simulink model "ev-pmsm-foc-model"  (R2025a)
settings: Solver=VariableStepAuto  StartTime=0.0  StopTime=10  RelTol=1e-3
undefined symbols (not defined in the file): J_m, K_d, k_g, Ki, Ki_s, Kp, Kp_s, L, lambda, p, R, r_w, T_rr
libraries: eeTransforms x4, slpidlib x3
settings Model: Creator=MEET  LastModifiedBy=MEET
settings SolverCC: ZeroCrossAlgorithm=Adaptive
settings DebuggingCC: IgnoredZcDiagnostic=none

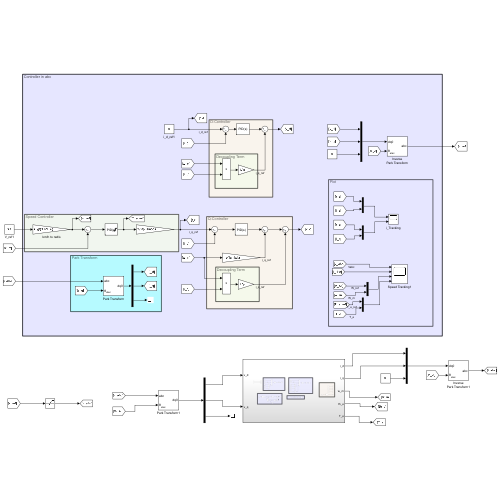
[thumbnail: Simulink's stored preview of the top-level diagram]
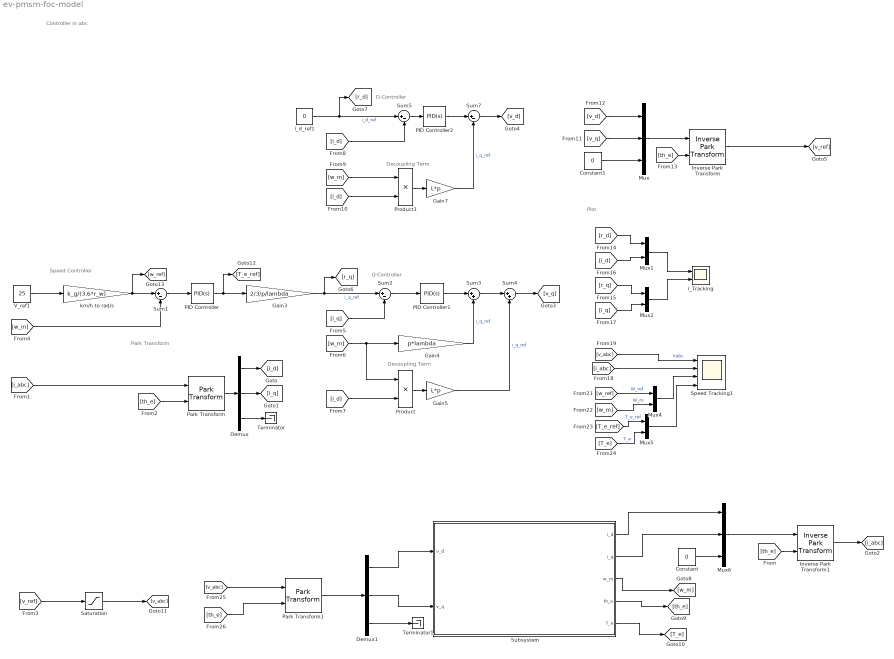
== system ev-pmsm-foc-model ==
  note: Controller in abc
  note: D-Controller
  note: Park Transform
  note: Decoupling Term
  note: Plot
  note: Decoupling Term
  note: Speed Controller
  note: Q-Controller
  Constant : Constant  Value=0
  Constant1 : Constant  Value=0
  Demux : Demux  Outputs=3
  Demux1 : Demux  Outputs=3
  Gain3 : Gain  Gain=2/3/p/lambda
  Gain4 : Gain  Gain=p*lambda
  Gain5 : Gain  Gain=L*p
  Gain7 : Gain  Gain=L*p
  Inverse Park Transform : eeTransforms/Inverse Park Transform  AxisAlignment=D-axis  PowerInvariant=off
      settings: LibrarySourceBlock=|
      | ee_sl_lib/Mathematical
      | Transforms/Inverse
      | Park Transform
  Inverse Park Transform1 : eeTransforms/Inverse Park Transform  AxisAlignment=D-axis  PowerInvariant=off
      settings: LibrarySourceBlock=|
      | ee_sl_lib/Mathematical
      | Transforms/Inverse
      | Park Transform
  Mux : Mux  Inputs=3
  Mux{1..2,4..5} (4 alike) : Mux  Inputs=2
  Mux6 : Mux  Inputs=3
  PID Controller : slpidlib/PID Controller  Controller=PID  Form=Parallel  TimeDomain=Continuous-time  UseExternalTs=off  SampleTime=-1  IntegratorMethod=Forward Euler  FilterMethod=Forward Euler  ControllerParametersSource=internal  P=Kp_s  I=Ki_s  UseKiTs=off  D=0  UseExternalDerivativeSource=off  N=100  UseFilter=on  TunerSelectOption=Transfer Function Based (PID Tuner App)  InitialConditionSource=internal  InitialConditionForIntegrator=0  InitialConditionForFilter=0  DifferentiatorICPrevScaledInput=0  ExternalReset=none  TrackingMode=off  Kt=1  LimitOutput=on  SatLimitsSource=internal  UpperSaturationLimit=108  LowerSaturationLimit=-108  LinearizeAsGain=on  AntiWindupMode=clamping  Kb=1  LimitIntegrator=off  UpperIntegratorSaturationLimit=inf  LowerIntegratorSaturationLimit=-inf  POutMin=[]  POutMax=[]  IOutMin=[]  IOutMax=[]  DOutMin=[]  DOutMax=[]  NOutMin=[]  NOutMax=[]  SumOutMin=[]  SumOutMax=[]  SaturationOutMin=[]  SaturationOutMax=[]  PParamMin=[]  PParamMax=[]  IParamMin=[]  IParamMax=[]  DParamMin=[]  DParamMax=[]  NParamMin=[]  NParamMax=[]  KbParamMin=[]  KbParamMax=[]  KtParamMin=[]  KtParamMax=[]  KbOutMin=[]  KbOutMax=[]  KtOutMin=[]  KtOutMax=[]  IntegratorOutMin=[]  IntegratorOutMax=[]  FilterOutMin=[]  FilterOutMax=[]  SumI1OutMin=[]  SumI1OutMax=[]  SumI2OutMin=[]  SumI2OutMax=[]  SumI3OutMin=[]  SumI3OutMax=[]  SumI4OutMin=[]  SumI4OutMax=[]  SumDOutMin=[]  SumDOutMax=[]  DifferentiatorOutMin=[]  DifferentiatorOutMax=[]  FilterDiffOutCoefMin=[]  FilterDiffOutCoefMax=[]  ReciprocalOutMin=[]  ReciprocalOutMax=[]  SumDenOutMin=[]  SumDenOutMax=[]  SumNumOutMin=[]  SumNumOutMax=[]  DivideOutMin=[]  DivideOutMax=[]  UdiffTsProdOutMin=[]  UdiffTsProdOutMax=[]  NTsProdOutMin=[]  NTsProdOutMax=[]  UintegralTsProdOutMin=[]  UintegralTsProdOutMax=[]  UngainTsProdOutMin=[]  UngainTsProdOutMax=[]  ClampingZeroOutDataTypeStr=Inherit: Inherit via back propagation  ClampingZeroOutMin=[]  ClampingZeroOutMax=[]  FilterDenConstantOutDataTypeStr=Inherit: Inherit via back propagation  FilterDenConstantOutMin=[]  FilterDenConstantOutMax=[]  PCopyOutDataTypeStr=Inherit: Inherit via back propagation  PCopyOutMin=[]  PCopyOutMax=[]  NCopyOutDataTypeStr=Inherit: Inherit via back propagation  NCopyOutMin=[]  NCopyOutMax=[]  IntegratorContinuousStateAttributes=''  IntegratorStateMustResolveToSignalObject=off  IntegratorRTWStateStorageClass=Auto  FilterContinuousStateAttributes=''  FilterStateMustResolveToSignalObject=off  FilterRTWStateStorageClass=Auto  ParallelPVariant=InternalParameters  IdealPVariant=Disabled  IVariant=InternalParameters  DVariant=InternalParameters  IntegratorVariant=Continuous  SatVariant=Enabled  AWVariant=ContClampingParallel  PCopyVariant=Disabled  TRVariant=Disabled  FdbkBlocksVariant=Forward  IdealPFdbkVariant=Disabled  SatFdbkVariant=Disabled  DerivativeFilterVariant=ContFilter  NVariant=InternalParameters  NCopyVariant=Disabled  FilterICVariant=InternalICsFilter  IntegratorICVariant=InternalICs  ExternalResetVariant=Disabled  TRSumVariant=Passthrough  SumFdbkVariant=Disabled  SumVariant=Sum_PID  TsampFilterVariant=InternalTs  TsampNgainVariant=Passthrough  TsampIntegralVariant=Disabled_SignalSpec  ExternalSaturationOutDataTypeStr=Inherit: Same as second input  DerivativeSourceVariant=ErrorSignal  PreIntVariant=InternalPreInt
  PID Controller1 : slpidlib/PID Controller  Controller=PID  Form=Parallel  TimeDomain=Continuous-time  UseExternalTs=off  SampleTime=-1  IntegratorMethod=Forward Euler  FilterMethod=Forward Euler  ControllerParametersSource=internal  P=Kp  I=Ki  UseKiTs=off  D=0  UseExternalDerivativeSource=off  N=100  UseFilter=on  TunerSelectOption=Transfer Function Based (PID Tuner App)  InitialConditionSource=internal  InitialConditionForIntegrator=0  InitialConditionForFilter=0  DifferentiatorICPrevScaledInput=0  ExternalReset=none  TrackingMode=off  Kt=1  LimitOutput=off  SatLimitsSource=internal  UpperSaturationLimit=inf  LowerSaturationLimit=-inf  LinearizeAsGain=on  AntiWindupMode=none  Kb=1  LimitIntegrator=off  UpperIntegratorSaturationLimit=inf  LowerIntegratorSaturationLimit=-inf  POutMin=[]  POutMax=[]  IOutMin=[]  IOutMax=[]  DOutMin=[]  DOutMax=[]  NOutMin=[]  NOutMax=[]  SumOutMin=[]  SumOutMax=[]  SaturationOutMin=[]  SaturationOutMax=[]  PParamMin=[]  PParamMax=[]  IParamMin=[]  IParamMax=[]  DParamMin=[]  DParamMax=[]  NParamMin=[]  NParamMax=[]  KbParamMin=[]  KbParamMax=[]  KtParamMin=[]  KtParamMax=[]  KbOutMin=[]  KbOutMax=[]  KtOutMin=[]  KtOutMax=[]  IntegratorOutMin=[]  IntegratorOutMax=[]  FilterOutMin=[]  FilterOutMax=[]  SumI1OutMin=[]  SumI1OutMax=[]  SumI2OutMin=[]  SumI2OutMax=[]  SumI3OutMin=[]  SumI3OutMax=[]  SumI4OutMin=[]  SumI4OutMax=[]  SumDOutMin=[]  SumDOutMax=[]  DifferentiatorOutMin=[]  DifferentiatorOutMax=[]  FilterDiffOutCoefMin=[]  FilterDiffOutCoefMax=[]  ReciprocalOutMin=[]  ReciprocalOutMax=[]  SumDenOutMin=[]  SumDenOutMax=[]  SumNumOutMin=[]  SumNumOutMax=[]  DivideOutMin=[]  DivideOutMax=[]  UdiffTsProdOutMin=[]  UdiffTsProdOutMax=[]  NTsProdOutMin=[]  NTsProdOutMax=[]  UintegralTsProdOutMin=[]  UintegralTsProdOutMax=[]  UngainTsProdOutMin=[]  UngainTsProdOutMax=[]  ClampingZeroOutDataTypeStr=Inherit: Inherit via back propagation  ClampingZeroOutMin=[]  ClampingZeroOutMax=[]  FilterDenConstantOutDataTypeStr=Inherit: Inherit via back propagation  FilterDenConstantOutMin=[]  FilterDenConstantOutMax=[]  PCopyOutDataTypeStr=Inherit: Inherit via back propagation  PCopyOutMin=[]  PCopyOutMax=[]  NCopyOutDataTypeStr=Inherit: Inherit via back propagation  NCopyOutMin=[]  NCopyOutMax=[]  IntegratorContinuousStateAttributes=''  IntegratorStateMustResolveToSignalObject=off  IntegratorRTWStateStorageClass=Auto  FilterContinuousStateAttributes=''  FilterStateMustResolveToSignalObject=off  FilterRTWStateStorageClass=Auto  ParallelPVariant=InternalParameters  IdealPVariant=Disabled  IVariant=InternalParameters  DVariant=InternalParameters  IntegratorVariant=Continuous  SatVariant=Disabled  AWVariant=Passthrough  PCopyVariant=Disabled  TRVariant=Disabled  FdbkBlocksVariant=Forward  IdealPFdbkVariant=Disabled  SatFdbkVariant=Disabled  DerivativeFilterVariant=ContFilter  NVariant=InternalParameters  NCopyVariant=Disabled  FilterICVariant=InternalICsFilter  IntegratorICVariant=InternalICs  ExternalResetVariant=Disabled  TRSumVariant=Passthrough  SumFdbkVariant=Disabled  SumVariant=Sum_PID  TsampFilterVariant=InternalTs  TsampNgainVariant=Passthrough  TsampIntegralVariant=Disabled_SignalSpec  ExternalSaturationOutDataTypeStr=Inherit: Same as second input  DerivativeSourceVariant=ErrorSignal  PreIntVariant=InternalPreInt
  PID Controller2 : slpidlib/PID Controller  Controller=PID  Form=Parallel  TimeDomain=Continuous-time  UseExternalTs=off  SampleTime=-1  IntegratorMethod=Forward Euler  FilterMethod=Forward Euler  ControllerParametersSource=internal  P=Kp  I=Ki  UseKiTs=off  D=0  UseExternalDerivativeSource=off  N=100  UseFilter=on  TunerSelectOption=Transfer Function Based (PID Tuner App)  InitialConditionSource=internal  InitialConditionForIntegrator=0  InitialConditionForFilter=0  DifferentiatorICPrevScaledInput=0  ExternalReset=none  TrackingMode=off  Kt=1  LimitOutput=off  SatLimitsSource=internal  UpperSaturationLimit=inf  LowerSaturationLimit=-inf  LinearizeAsGain=on  AntiWindupMode=none  Kb=1  LimitIntegrator=off  UpperIntegratorSaturationLimit=inf  LowerIntegratorSaturationLimit=-inf  POutMin=[]  POutMax=[]  IOutMin=[]  IOutMax=[]  DOutMin=[]  DOutMax=[]  NOutMin=[]  NOutMax=[]  SumOutMin=[]  SumOutMax=[]  SaturationOutMin=[]  SaturationOutMax=[]  PParamMin=[]  PParamMax=[]  IParamMin=[]  IParamMax=[]  DParamMin=[]  DParamMax=[]  NParamMin=[]  NParamMax=[]  KbParamMin=[]  KbParamMax=[]  KtParamMin=[]  KtParamMax=[]  KbOutMin=[]  KbOutMax=[]  KtOutMin=[]  KtOutMax=[]  IntegratorOutMin=[]  IntegratorOutMax=[]  FilterOutMin=[]  FilterOutMax=[]  SumI1OutMin=[]  SumI1OutMax=[]  SumI2OutMin=[]  SumI2OutMax=[]  SumI3OutMin=[]  SumI3OutMax=[]  SumI4OutMin=[]  SumI4OutMax=[]  SumDOutMin=[]  SumDOutMax=[]  DifferentiatorOutMin=[]  DifferentiatorOutMax=[]  FilterDiffOutCoefMin=[]  FilterDiffOutCoefMax=[]  ReciprocalOutMin=[]  ReciprocalOutMax=[]  SumDenOutMin=[]  SumDenOutMax=[]  SumNumOutMin=[]  SumNumOutMax=[]  DivideOutMin=[]  DivideOutMax=[]  UdiffTsProdOutMin=[]  UdiffTsProdOutMax=[]  NTsProdOutMin=[]  NTsProdOutMax=[]  UintegralTsProdOutMin=[]  UintegralTsProdOutMax=[]  UngainTsProdOutMin=[]  UngainTsProdOutMax=[]  ClampingZeroOutDataTypeStr=Inherit: Inherit via back propagation  ClampingZeroOutMin=[]  ClampingZeroOutMax=[]  FilterDenConstantOutDataTypeStr=Inherit: Inherit via back propagation  FilterDenConstantOutMin=[]  FilterDenConstantOutMax=[]  PCopyOutDataTypeStr=Inherit: Inherit via back propagation  PCopyOutMin=[]  PCopyOutMax=[]  NCopyOutDataTypeStr=Inherit: Inherit via back propagation  NCopyOutMin=[]  NCopyOutMax=[]  IntegratorContinuousStateAttributes=''  IntegratorStateMustResolveToSignalObject=off  IntegratorRTWStateStorageClass=Auto  FilterContinuousStateAttributes=''  FilterStateMustResolveToSignalObject=off  FilterRTWStateStorageClass=Auto  ParallelPVariant=InternalParameters  IdealPVariant=Disabled  IVariant=InternalParameters  DVariant=InternalParameters  IntegratorVariant=Continuous  SatVariant=Disabled  AWVariant=Passthrough  PCopyVariant=Disabled  TRVariant=Disabled  FdbkBlocksVariant=Forward  IdealPFdbkVariant=Disabled  SatFdbkVariant=Disabled  DerivativeFilterVariant=ContFilter  NVariant=InternalParameters  NCopyVariant=Disabled  FilterICVariant=InternalICsFilter  IntegratorICVariant=InternalICs  ExternalResetVariant=Disabled  TRSumVariant=Passthrough  SumFdbkVariant=Disabled  SumVariant=Sum_PID  TsampFilterVariant=InternalTs  TsampNgainVariant=Passthrough  TsampIntegralVariant=Disabled_SignalSpec  ExternalSaturationOutDataTypeStr=Inherit: Same as second input  DerivativeSourceVariant=ErrorSignal  PreIntVariant=InternalPreInt
  Park Transform : eeTransforms/Park Transform  AxisAlignment=D-axis  PowerInvariant=off
      settings: LibrarySourceBlock=|
      | ee_sl_lib/Mathematical
      | Transforms/Park Transform
  Park Transform1 : eeTransforms/Park Transform  AxisAlignment=D-axis  PowerInvariant=off
      settings: LibrarySourceBlock=|
      | ee_sl_lib/Mathematical
      | Transforms/Park Transform
  Product : Product
  Product1 : Product
  Saturation : Saturate  UpperLimit=150  LowerLimit=-150
  Speed Tracking1 : Scope  NumInputPorts=4
      settings: ActiveDisplayYMinimum=-125  ActiveDisplayYMaximum=125  DataLoggingVariableName=ScopeData2
  Subsystem : Subsystem
  Sum{1..2,5,7} (4 alike) : Sum  Inputs=|+-
  Sum3 : Sum  Inputs=|++
  Sum4 : Sum  Inputs=|++
  Terminator : Terminator
  Terminator1 : Terminator
  V_ref1 : Constant  Value=25
  i_Tracking : Scope  NumInputPorts=2
      settings: ActiveDisplayYMinimum=-327.57721760739042  ActiveDisplayYMaximum=215.31505153767358
  i_d_ref1 : Constant  Value=0
  km/h to rad/s : Gain  Gain=k_g/(3.6*r_w)
  wires:
  Sum7/1 -> [v_d]
  Demux/3 -> Terminator/1
  [w_m] -> Mux4/2  "W_m"
  km/h to rad/s/1 -> [w_ref], Sum1/1
  [T_e] -> Mux5/2  "T_e"
  [w_m] -> Product/1, Gain4/1
  [i_d] -> Product1/2
  i_d_ref1/1 -> [r_d], Sum5/1  "i_d_ref"
  Mux4/1 -> Speed Tracking1/3
  [v_q] -> Mux/2
  [r_q] -> Mux2/1
  Gain4/1 -> Sum3/2  "i_q_ref"
  [i_q] -> Mux2/2
  Constant1/1 -> Mux/3
  [i_d] -> Sum5/2
  [i_q] -> Sum2/2
  Mux/1 -> Inverse Park Transform/1
  V_ref1/1 -> km/h to rad/s/1
  [T_e_ref] -> Mux5/1  "T_e_ref"
  Demux/2 -> [i_q]
  Mux2/1 -> i_Tracking/2
  [i_abc] -> Park Transform/1
  [w_m] -> Product1/1
  [v_abc] -> Speed Tracking1/1  "Vabc"
  Gain3/1 -> Sum2/1, [r_q]  "i_q_ref"
  Mux5/1 -> Speed Tracking1/4
  [th_e] -> Inverse Park Transform/2
  Mux1/1 -> i_Tracking/1
  Gain7/1 -> Sum7/2  "i_q_ref"
  Park Transform/1 -> Demux/1
  PID Controller2/1 -> Sum7/1
  [v_d] -> Mux/1
  Sum4/1 -> [v_q]
  Product1/1 -> Gain7/1
  Demux/1 -> [i_d]
  Sum1/1 -> PID Controller/1
  Sum3/1 -> Sum4/1
  [w_ref] -> Mux4/1  "W_ref"
  Gain5/1 -> Sum4/2  "i_q_ref"
  [i_d] -> Mux1/2
  [th_e] -> Park Transform/2
  Sum5/1 -> PID Controller2/1
  Inverse Park Transform/1 -> [v_ref]
  PID Controller1/1 -> Sum3/1
  Sum2/1 -> PID Controller1/1
  [i_d] -> Product/2
  Product/1 -> Gain5/1
  [r_d] -> Mux1/1
  PID Controller/1 -> [T_e_ref], Gain3/1
  [w_m] -> Sum1/2
  [v_abc] -> Park Transform1/1
  [th_e] -> Park Transform1/2
  Park Transform1/1 -> Demux1/1
  Demux1/3 -> Terminator1/1
  Demux1/1 -> Subsystem/1(v_d)
  Demux1/2 -> Subsystem/2(v_q)
  Subsystem/3(w_m) -> [w_m]
  Subsystem/5(T_e) -> [T_e]
  Subsystem/4(th_e) -> [th_e]
  Constant/1 -> Mux6/3
  Subsystem/2(i_q) -> Mux6/2
  Subsystem/1(i_d) -> Mux6/1
  Mux6/1 -> Inverse Park Transform1/1
  [th_e] -> Inverse Park Transform1/2
  Inverse Park Transform1/1 -> [i_abc]
  [v_ref] -> Saturation/1
  Saturation/1 -> [v_abc]
  [i_abc] -> Speed Tracking1/2

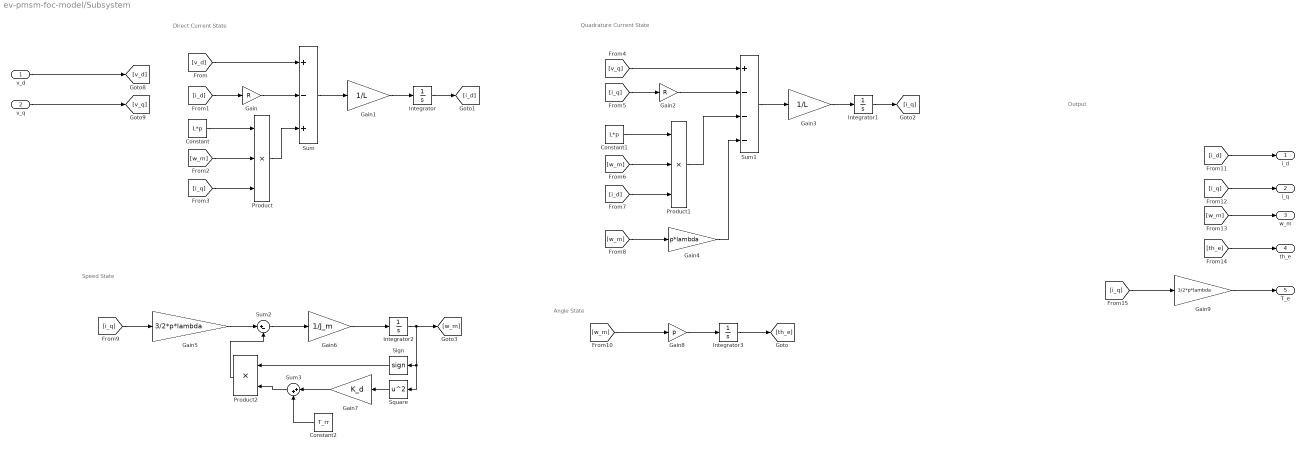
== system ev-pmsm-foc-model/Subsystem ==
  note: Output
  note: Angle State
  note: Speed State
  note: Quadrature Current State
  note: Direct Current State
  v_d : Inport
  v_q : Inport  Port=2
  Constant : Constant  Value=L*p
  Constant1 : Constant  Value=L*p
  Constant2 : Constant  Value=T_rr
  Gain : Gain  Gain=R
  Gain1 : Gain  Gain=1/L
  Gain2 : Gain  Gain=R
  Gain3 : Gain  Gain=1/L
  Gain4 : Gain  Gain=p*lambda
  Gain5 : Gain  Gain=3/2*p*lambda
  Gain6 : Gain  Gain=1/J_m
  Gain7 : Gain  Gain=K_d
  Gain8 : Gain  Gain=p
  Gain9 : Gain  Gain=3/2*p*lambda
  Integrator{,1..3} (4 alike) : Integrator
  Product : Product  Inputs=3
  Product1 : Product  Inputs=3
  Product2 : Product
  Sign : Signum
  Square : Math  Operator=square
  Sum : Sum  Inputs=+-+
  Sum1 : Sum  Inputs=+---
  Sum2 : Sum  Inputs=|+-
  Sum3 : Sum  Inputs=|++
  i_d : Outport
  i_q : Outport  Port=2
  w_m : Outport  Port=3
  th_e : Outport  Port=4
  T_e : Outport  Port=5
  wires:
  v_q/1 -> [v_q]
  v_d/1 -> [v_d]
  Constant/1 -> Product/1
  [w_m] -> Product/2
  [i_q] -> Product/3
  Product/1 -> Sum/3
  [i_d] -> Gain/1
  Gain/1 -> Sum/2
  [v_d] -> Sum/1
  Sum/1 -> Gain1/1
  Gain1/1 -> Integrator/1
  Integrator/1 -> [i_d]
  Sum1/1 -> Gain3/1
  Gain3/1 -> Integrator1/1
  Product1/1 -> Sum1/3
  [w_m] -> Product1/2
  Gain2/1 -> Sum1/2
  Constant1/1 -> Product1/1
  Integrator1/1 -> [i_q]
  [v_q] -> Sum1/1
  [i_q] -> Gain2/1
  [i_d] -> Product1/3
  [w_m] -> Gain4/1
  Gain4/1 -> Sum1/4
  [i_q] -> Gain5/1
  Gain5/1 -> Sum2/1
  Sum2/1 -> Gain6/1
  Gain6/1 -> Integrator2/1
  Integrator2/1 -> [w_m], Sign/1, Square/1
  Square/1 -> Gain7/1
  Sum3/1 -> Product2/2
  Sign/1 -> Product2/1
  Gain7/1 -> Sum3/1
  Constant2/1 -> Sum3/2
  [w_m] -> Gain8/1
  Gain8/1 -> Integrator3/1
  Integrator3/1 -> [th_e]
  [i_q] -> Gain9/1
  Gain9/1 -> T_e/1
  [th_e] -> th_e/1
  [w_m] -> w_m/1
  [i_q] -> i_q/1
  [i_d] -> i_d/1
  Product2/1 -> Sum2/2
